simulink library "Susp_Components"  (R2026a)
settings: Solver=VariableStepAuto
undefined symbols (not defined in the file): clr_conn_links, clr_conn_rod, clr_link, clr_uaf, hp_in_f_ua, hp_out_f_ua, hp_shock_bot, hp_shock_botL, hp_shock_top, hp_shock_topL, hp_steerlink_out, hp_steerlink_outL, hp_upr_axle, hp_upr_axleL, hp_upr_drag, hp_upr_dragL, hp_wattsl_body, hp_wattsl_pivot, hp_wattsp_axle, hp_wattsu_body, hp_wattsu_pivot, hp_whl_ctr, hp_whl_ctrL, opc_conn_links, opc_conn_rod, opc_link, opc_uaf, radius_link, radius_uaf, size_conn_links, size_conn_rod, Susp, uaf_mass, upr_mass, Visual, wattsl_mass, wattsp_mass, wattsu_mass, X, Y, Z
libraries: sm_lib x32, Suspension_Utilities x10, Linkage_Shock x4, nesl_utility x3, $bdroot x2
(part 2 of 2)

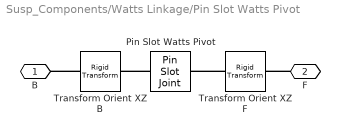
== system Susp_Components/Watts Linkage/Pin Slot Watts Pivot ==
  Pin Slot Watts Pivot : sm_lib/Joints/Pin Slot Joint  JointMode=Normal  CompositeWrenchDir=FollowerOnBase  CompositeWrenchFrame=BaseFrame  SenseConstraintForce=off  SenseConstraintTorque=off  SenseTotalForce=off  SenseTotalTorque=off  PxPositionTargetSpecify=off  PxPositionTargetPriority=High  PxPositionTargetValue=0  PxPositionTargetValueUnits=m  PxVelocityTargetSpecify=off  PxVelocityTargetPriority=High  PxVelocityTargetValue=0  PxVelocityTargetValueUnits=m/s  PxEquilibriumPosition=0  PxEquilibriumPositionUnits=m  PxSpringStiffness=0  PxSpringStiffnessUnits=N/m  PxDampingCoefficient=0  PxDampingCoefficientUnits=N/(m/s)  PxLowerLimitSpecify=off  PxLowerLimitBound=-1  PxLowerLimitBoundUnits=m  PxLowerLimitStiffness=1e6  PxLowerLimitStiffnessUnits=N/m  PxLowerLimitDamping=1e3  PxLowerLimitDampingUnits=N/(m/s)  PxLowerLimitTransitionRegionWidth=1e-4  PxLowerLimitTransitionRegionWidthUnits=m  PxUpperLimitSpecify=off  PxUpperLimitBound=1  PxUpperLimitBoundUnits=m  PxUpperLimitStiffness=1e6  PxUpperLimitStiffnessUnits=N/m  PxUpperLimitDamping=1e3  PxUpperLimitDampingUnits=N/(m/s)  PxUpperLimitTransitionRegionWidth=1e-4  PxUpperLimitTransitionRegionWidthUnits=m  PxTorqueActuationMode=NoTorque  PxMotionActuationMode=ComputedMotion  PxSensePosition=off  PxSenseVelocity=off  PxSenseAcceleration=off  PxSenseTorqueForce=off  PxSenseLowerLimitTorqueForce=off  PxSenseUpperLimitTorqueForce=off  RzPositionTargetSpecify=off  RzPositionTargetPriority=High  RzPositionTargetValue=0  RzPositionTargetValueUnits=deg  RzVelocityTargetSpecify=off  RzVelocityTargetPriority=High  RzVelocityTargetValue=0  RzVelocityTargetValueUnits=deg/s  RzEquilibriumPosition=0  RzEquilibriumPositionUnits=deg  RzSpringStiffness=0  RzSpringStiffnessUnits=N*m/deg  RzDampingCoefficient=0  RzDampingCoefficientUnits=N*m/(deg/s)  RzLowerLimitSpecify=off  RzLowerLimitBound=-90  RzLowerLimitBoundUnits=deg  RzLowerLimitStiffness=1e4  RzLowerLimitStiffnessUnits=N*m/deg  RzLowerLimitDamping=10  RzLowerLimitDampingUnits=N*m/(deg/s)  RzLowerLimitTransitionRegionWidth=0.1  RzLowerLimitTransitionRegionWidthUnits=deg  RzUpperLimitSpecify=off  RzUpperLimitBound=90  RzUpperLimitBoundUnits=deg  RzUpperLimitStiffness=1e4  RzUpperLimitStiffnessUnits=N*m/deg  RzUpperLimitDamping=10  RzUpperLimitDampingUnits=N*m/(deg/s)  RzUpperLimitTransitionRegionWidth=0.1  RzUpperLimitTransitionRegionWidthUnits=deg  RzTorqueActuationMode=NoTorque  RzMotionActuationMode=ComputedMotion  RzSensePosition=off  RzSenseVelocity=off  RzSenseAcceleration=off  RzSenseTorqueForce=off  RzSenseLowerLimitTorqueForce=off  RzSenseUpperLimitTorqueForce=off
  Transform Orient XZ B : sm_lib/Frames and Transforms/Rigid Transform  RotationMethod=AlignedAxes  FollAlignAxisA=+Z  BaseAlignAxisA=+X  FollAlignAxisB=+X  BaseAlignAxisB=+Y  RotationStandardAxis=+Z  RotationAngle=0.0  RotationAngleUnits=deg  RotationArbitraryAxis=[0 0 1]  RotationSequenceAxes=FollowerAxes  RotationSequence=XYX  RotationSequenceAngles=[0 0 0]  RotationSequenceAnglesUnits=deg  RotationMatrix=[1 0 0; 0 1 0; 0 0 1]  Quaternion=[1 0 0 0]  TranslationMethod=None  TranslationCartesianOffset=[0 0 0]  TranslationCartesianOffsetUnits=m  TranslationStandardAxis=+Z  TranslationStandardOffset=0  TranslationStandardOffsetUnits=m  TranslationROffset=0  TranslationROffsetUnits=m  TranslationThetaOffset=0  TranslationThetaOffsetUnits=deg  TranslationZOffset=0  TranslationZOffsetUnits=m
  Transform Orient XZ F : sm_lib/Frames and Transforms/Rigid Transform  RotationMethod=AlignedAxes  FollAlignAxisA=+Z  BaseAlignAxisA=+X  FollAlignAxisB=+X  BaseAlignAxisB=+Y  RotationStandardAxis=+Z  RotationAngle=0.0  RotationAngleUnits=deg  RotationArbitraryAxis=[0 0 1]  RotationSequenceAxes=FollowerAxes  RotationSequence=XYX  RotationSequenceAngles=[0 0 0]  RotationSequenceAnglesUnits=deg  RotationMatrix=[1 0 0; 0 1 0; 0 0 1]  Quaternion=[1 0 0 0]  TranslationMethod=None  TranslationCartesianOffset=[0 0 0]  TranslationCartesianOffsetUnits=m  TranslationStandardAxis=+Z  TranslationStandardOffset=0  TranslationStandardOffsetUnits=m  TranslationROffset=0  TranslationROffsetUnits=m  TranslationThetaOffset=0  TranslationThetaOffsetUnits=deg  TranslationZOffset=0  TranslationZOffsetUnits=m
  B : PMIOPort  Side=Left
  F : PMIOPort  Port=2  Side=Right
  connections:
  Transform Orient XZ F/RConn1 -- Pin Slot Watts Pivot/RConn1
  Pin Slot Watts Pivot/LConn1 -- Transform Orient XZ B/RConn1
  Transform Orient XZ B/LConn1 -- B/RConn1
  F/RConn1 -- Transform Orient XZ F/LConn1

== system Susp_Components/Watts Linkage/Universal Pivot Upper ==
  Transform Orient Z B : sm_lib/Frames and Transforms/Rigid Transform  RotationMethod=StandardAxis  FollAlignAxisA=+X  BaseAlignAxisA=+Y  FollAlignAxisB=+Y  BaseAlignAxisB=+Z  RotationStandardAxis=+X  RotationAngle=90  RotationAngleUnits=deg  RotationArbitraryAxis=[0 0 1]  RotationSequenceAxes=FollowerAxes  RotationSequence=XYX  RotationSequenceAngles=[0 0 0]  RotationSequenceAnglesUnits=deg  RotationMatrix=[1 0 0;0 1 0;0 0 1]  Quaternion=[1 0 0 0]  TranslationMethod=None  TranslationCartesianOffset=[0 0 0]  TranslationCartesianOffsetUnits=m  TranslationStandardAxis=+Z  TranslationStandardOffset=0  TranslationStandardOffsetUnits=m  TranslationROffset=0  TranslationROffsetUnits=m  TranslationThetaOffset=0  TranslationThetaOffsetUnits=deg  TranslationZOffset=0  TranslationZOffsetUnits=m
  Transform Orient Z F : sm_lib/Frames and Transforms/Rigid Transform  RotationMethod=StandardAxis  FollAlignAxisA=+X  BaseAlignAxisA=+Y  FollAlignAxisB=+Y  BaseAlignAxisB=+Z  RotationStandardAxis=+X  RotationAngle=90  RotationAngleUnits=deg  RotationArbitraryAxis=[0 0 1]  RotationSequenceAxes=FollowerAxes  RotationSequence=XYX  RotationSequenceAngles=[0 0 0]  RotationSequenceAnglesUnits=deg  RotationMatrix=[1 0 0;0 1 0;0 0 1]  Quaternion=[1 0 0 0]  TranslationMethod=None  TranslationCartesianOffset=[0 0 0]  TranslationCartesianOffsetUnits=m  TranslationStandardAxis=+Z  TranslationStandardOffset=0  TranslationStandardOffsetUnits=m  TranslationROffset=0  TranslationROffsetUnits=m  TranslationThetaOffset=0  TranslationThetaOffsetUnits=deg  TranslationZOffset=0  TranslationZOffsetUnits=m
  Universal Pivot Upper : sm_lib/Joints/Universal Joint  JointMode=Normal  CompositeWrenchDir=FollowerOnBase  CompositeWrenchFrame=BaseFrame  SenseConstraintForce=off  SenseConstraintTorque=off  SenseTotalForce=off  SenseTotalTorque=off  RxPositionTargetSpecify=off  RxPositionTargetPriority=High  RxPositionTargetValue=0  RxPositionTargetValueUnits=deg  RxVelocityTargetSpecify=off  RxVelocityTargetPriority=High  RxVelocityTargetValue=0  RxVelocityTargetValueUnits=deg/s  RxEquilibriumPosition=0  RxEquilibriumPositionUnits=deg  RxSpringStiffness=0  RxSpringStiffnessUnits=N*m/deg  RxDampingCoefficient=0  RxDampingCoefficientUnits=N*m/(deg/s)  RxLowerLimitSpecify=off  RxLowerLimitBound=-90  RxLowerLimitBoundUnits=deg  RxLowerLimitStiffness=1e4  RxLowerLimitStiffnessUnits=N*m/deg  RxLowerLimitDamping=10  RxLowerLimitDampingUnits=N*m/(deg/s)  RxLowerLimitTransitionRegionWidth=0.1  RxLowerLimitTransitionRegionWidthUnits=deg  RxUpperLimitSpecify=off  RxUpperLimitBound=90  RxUpperLimitBoundUnits=deg  RxUpperLimitStiffness=1e4  RxUpperLimitStiffnessUnits=N*m/deg  RxUpperLimitDamping=10  RxUpperLimitDampingUnits=N*m/(deg/s)  RxUpperLimitTransitionRegionWidth=0.1  RxUpperLimitTransitionRegionWidthUnits=deg  RxTorqueActuationMode=NoTorque  RxMotionActuationMode=ComputedMotion  RxSensePosition=off  RxSenseVelocity=off  RxSenseAcceleration=off  RxSenseTorqueForce=off  RxSenseLowerLimitTorqueForce=off  RxSenseUpperLimitTorqueForce=off  RyPositionTargetSpecify=off  RyPositionTargetPriority=High  RyPositionTargetValue=0  RyPositionTargetValueUnits=deg  RyVelocityTargetSpecify=off  RyVelocityTargetPriority=High  RyVelocityTargetValue=0  RyVelocityTargetValueUnits=deg/s  RyEquilibriumPosition=0  RyEquilibriumPositionUnits=deg  RySpringStiffness=0  RySpringStiffnessUnits=N*m/deg  RyDampingCoefficient=0  RyDampingCoefficientUnits=N*m/(deg/s)  RyLowerLimitSpecify=off  RyLowerLimitBound=-90  RyLowerLimitBoundUnits=deg  RyLowerLimitStiffness=1e4  RyLowerLimitStiffnessUnits=N*m/deg  RyLowerLimitDamping=10  RyLowerLimitDampingUnits=N*m/(deg/s)  RyLowerLimitTransitionRegionWidth=0.1  RyLowerLimitTransitionRegionWidthUnits=deg  RyUpperLimitSpecify=off  RyUpperLimitBound=90  RyUpperLimitBoundUnits=deg  RyUpperLimitStiffness=1e4  RyUpperLimitStiffnessUnits=N*m/deg  RyUpperLimitDamping=10  RyUpperLimitDampingUnits=N*m/(deg/s)  RyUpperLimitTransitionRegionWidth=0.1  RyUpperLimitTransitionRegionWidthUnits=deg  RyTorqueActuationMode=NoTorque  RyMotionActuationMode=ComputedMotion  RySensePosition=off  RySenseVelocity=off  RySenseAcceleration=off  RySenseTorqueForce=off  RySenseLowerLimitTorqueForce=off  RySenseUpperLimitTorqueForce=off
  B : PMIOPort  Side=Left
  F : PMIOPort  Port=2  Side=Right
  connections:
  Transform Orient Z B/RConn1 -- Universal Pivot Upper/LConn1
  Transform Orient Z B/LConn1 -- B/RConn1
  Transform Orient Z F/RConn1 -- Universal Pivot Upper/RConn1
  Transform Orient Z F/LConn1 -- F/RConn1

== system Susp_Components/Watts Linkage/Universal Watts Pivot Lower ==
  Transform Orient Z B : sm_lib/Frames and Transforms/Rigid Transform  RotationMethod=StandardAxis  FollAlignAxisA=+X  BaseAlignAxisA=+Y  FollAlignAxisB=+Y  BaseAlignAxisB=+Z  RotationStandardAxis=+X  RotationAngle=90  RotationAngleUnits=deg  RotationArbitraryAxis=[0 0 1]  RotationSequenceAxes=FollowerAxes  RotationSequence=XYX  RotationSequenceAngles=[0 0 0]  RotationSequenceAnglesUnits=deg  RotationMatrix=[1 0 0;0 1 0;0 0 1]  Quaternion=[1 0 0 0]  TranslationMethod=None  TranslationCartesianOffset=[0 0 0]  TranslationCartesianOffsetUnits=m  TranslationStandardAxis=+Z  TranslationStandardOffset=0  TranslationStandardOffsetUnits=m  TranslationROffset=0  TranslationROffsetUnits=m  TranslationThetaOffset=0  TranslationThetaOffsetUnits=deg  TranslationZOffset=0  TranslationZOffsetUnits=m
  Transform Orient Z F : sm_lib/Frames and Transforms/Rigid Transform  RotationMethod=StandardAxis  FollAlignAxisA=+X  BaseAlignAxisA=+Y  FollAlignAxisB=+Y  BaseAlignAxisB=+Z  RotationStandardAxis=+X  RotationAngle=90  RotationAngleUnits=deg  RotationArbitraryAxis=[0 0 1]  RotationSequenceAxes=FollowerAxes  RotationSequence=XYX  RotationSequenceAngles=[0 0 0]  RotationSequenceAnglesUnits=deg  RotationMatrix=[1 0 0;0 1 0;0 0 1]  Quaternion=[1 0 0 0]  TranslationMethod=None  TranslationCartesianOffset=[0 0 0]  TranslationCartesianOffsetUnits=m  TranslationStandardAxis=+Z  TranslationStandardOffset=0  TranslationStandardOffsetUnits=m  TranslationROffset=0  TranslationROffsetUnits=m  TranslationThetaOffset=0  TranslationThetaOffsetUnits=deg  TranslationZOffset=0  TranslationZOffsetUnits=m
  Universal Pivot Lower : sm_lib/Joints/Universal Joint  JointMode=Normal  CompositeWrenchDir=FollowerOnBase  CompositeWrenchFrame=BaseFrame  SenseConstraintForce=off  SenseConstraintTorque=off  SenseTotalForce=off  SenseTotalTorque=off  RxPositionTargetSpecify=off  RxPositionTargetPriority=High  RxPositionTargetValue=0  RxPositionTargetValueUnits=deg  RxVelocityTargetSpecify=off  RxVelocityTargetPriority=High  RxVelocityTargetValue=0  RxVelocityTargetValueUnits=deg/s  RxEquilibriumPosition=0  RxEquilibriumPositionUnits=deg  RxSpringStiffness=0  RxSpringStiffnessUnits=N*m/deg  RxDampingCoefficient=0  RxDampingCoefficientUnits=N*m/(deg/s)  RxLowerLimitSpecify=off  RxLowerLimitBound=-90  RxLowerLimitBoundUnits=deg  RxLowerLimitStiffness=1e4  RxLowerLimitStiffnessUnits=N*m/deg  RxLowerLimitDamping=10  RxLowerLimitDampingUnits=N*m/(deg/s)  RxLowerLimitTransitionRegionWidth=0.1  RxLowerLimitTransitionRegionWidthUnits=deg  RxUpperLimitSpecify=off  RxUpperLimitBound=90  RxUpperLimitBoundUnits=deg  RxUpperLimitStiffness=1e4  RxUpperLimitStiffnessUnits=N*m/deg  RxUpperLimitDamping=10  RxUpperLimitDampingUnits=N*m/(deg/s)  RxUpperLimitTransitionRegionWidth=0.1  RxUpperLimitTransitionRegionWidthUnits=deg  RxTorqueActuationMode=NoTorque  RxMotionActuationMode=ComputedMotion  RxSensePosition=off  RxSenseVelocity=off  RxSenseAcceleration=off  RxSenseTorqueForce=off  RxSenseLowerLimitTorqueForce=off  RxSenseUpperLimitTorqueForce=off  RyPositionTargetSpecify=off  RyPositionTargetPriority=High  RyPositionTargetValue=0  RyPositionTargetValueUnits=deg  RyVelocityTargetSpecify=off  RyVelocityTargetPriority=High  RyVelocityTargetValue=0  RyVelocityTargetValueUnits=deg/s  RyEquilibriumPosition=0  RyEquilibriumPositionUnits=deg  RySpringStiffness=0  RySpringStiffnessUnits=N*m/deg  RyDampingCoefficient=0  RyDampingCoefficientUnits=N*m/(deg/s)  RyLowerLimitSpecify=off  RyLowerLimitBound=-90  RyLowerLimitBoundUnits=deg  RyLowerLimitStiffness=1e4  RyLowerLimitStiffnessUnits=N*m/deg  RyLowerLimitDamping=10  RyLowerLimitDampingUnits=N*m/(deg/s)  RyLowerLimitTransitionRegionWidth=0.1  RyLowerLimitTransitionRegionWidthUnits=deg  RyUpperLimitSpecify=off  RyUpperLimitBound=90  RyUpperLimitBoundUnits=deg  RyUpperLimitStiffness=1e4  RyUpperLimitStiffnessUnits=N*m/deg  RyUpperLimitDamping=10  RyUpperLimitDampingUnits=N*m/(deg/s)  RyUpperLimitTransitionRegionWidth=0.1  RyUpperLimitTransitionRegionWidthUnits=deg  RyTorqueActuationMode=NoTorque  RyMotionActuationMode=ComputedMotion  RySensePosition=off  RySenseVelocity=off  RySenseAcceleration=off  RySenseTorqueForce=off  RySenseLowerLimitTorqueForce=off  RySenseUpperLimitTorqueForce=off
  B : PMIOPort  Side=Left
  F : PMIOPort  Port=2  Side=Right
  connections:
  Transform Orient Z F/LConn1 -- F/RConn1
  Transform Orient Z F/RConn1 -- Universal Pivot Lower/RConn1
  Transform Orient Z B/LConn1 -- B/RConn1
  Transform Orient Z B/RConn1 -- Universal Pivot Lower/LConn1

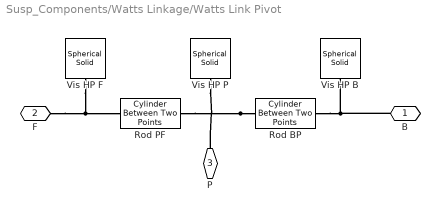
== system Susp_Components/Watts Linkage/Watts Link Pivot ==
  Rod BP : Suspension_Utilities/Cylinder Between Two Points  hp_b=hp_b.*[1 rhs_rod 1]  hp_f=hp_piv.*[1 rhs_rod 1]  Mass=rod_mass/2  clr_solid=clr_rod  opc_solid=opc_rod  rad_solid=radius_rod
  Rod PF : Suspension_Utilities/Cylinder Between Two Points  hp_b=hp_piv.*[1 rhs_rod 1]  hp_f=hp_f.*[1 rhs_rod 1]  Mass=rod_mass/2  clr_solid=clr_rod  opc_solid=opc_rod  rad_solid=radius_rod
  Vis HP B : sm_lib/Body Elements/Spherical Solid  SphereRadius=size_conn_rod  SphereRadiusUnits=m  ExportEntireGeometry=off  InertiaType=CalculateFromGeometry  BasedOnType=Density  Density=0  DensityUnits=kg/m^3  Mass=1  MassUnits=kg  CenterOfMass=[0 0 0]  CenterOfMassUnits=m  MomentsOfInertia=[1 1 1]  MomentsOfInertiaUnits=kg*m^2  ProductsOfInertia=[0 0 0]  ProductsOfInertiaUnits=kg*m^2  GraphicType=FromGeometry  MarkerShape=Sphere  MarkerSize=10  GraphicVisPropType=SimpleVisualProperties  GraphicDiffuseColor=clr_conn_rod  GraphicOpacity=opc_conn_rod  GraphicSpecularColor=[0.5 0.5 0.5 1.0]  GraphicAmbientColor=[0.15 0.15 0.15 1.0]  GraphicEmissiveColor=[0.0 0.0 0.0 1.0]  GraphicShininess=75  DoExposeReferenceFrame=on  SerializedFrames=<Frames/>
  Vis HP F : sm_lib/Body Elements/Spherical Solid  SphereRadius=size_conn_rod  SphereRadiusUnits=m  ExportEntireGeometry=off  InertiaType=CalculateFromGeometry  BasedOnType=Density  Density=0  DensityUnits=kg/m^3  Mass=1  MassUnits=kg  CenterOfMass=[0 0 0]  CenterOfMassUnits=m  MomentsOfInertia=[1 1 1]  MomentsOfInertiaUnits=kg*m^2  ProductsOfInertia=[0 0 0]  ProductsOfInertiaUnits=kg*m^2  GraphicType=FromGeometry  MarkerShape=Sphere  MarkerSize=10  GraphicVisPropType=SimpleVisualProperties  GraphicDiffuseColor=clr_conn_rod  GraphicOpacity=opc_conn_rod  GraphicSpecularColor=[0.5 0.5 0.5 1.0]  GraphicAmbientColor=[0.15 0.15 0.15 1.0]  GraphicEmissiveColor=[0.0 0.0 0.0 1.0]  GraphicShininess=75  DoExposeReferenceFrame=on  SerializedFrames=<Frames/>
  Vis HP P : sm_lib/Body Elements/Spherical Solid  SphereRadius=size_conn_rod  SphereRadiusUnits=m  ExportEntireGeometry=off  InertiaType=CalculateFromGeometry  BasedOnType=Density  Density=0  DensityUnits=kg/m^3  Mass=1  MassUnits=kg  CenterOfMass=[0 0 0]  CenterOfMassUnits=m  MomentsOfInertia=[1 1 1]  MomentsOfInertiaUnits=kg*m^2  ProductsOfInertia=[0 0 0]  ProductsOfInertiaUnits=kg*m^2  GraphicType=FromGeometry  MarkerShape=Sphere  MarkerSize=10  GraphicVisPropType=SimpleVisualProperties  GraphicDiffuseColor=clr_conn_rod  GraphicOpacity=opc_conn_rod  GraphicSpecularColor=[0.5 0.5 0.5 1.0]  GraphicAmbientColor=[0.15 0.15 0.15 1.0]  GraphicEmissiveColor=[0.0 0.0 0.0 1.0]  GraphicShininess=75  DoExposeReferenceFrame=on  SerializedFrames=<Frames/>
  B : PMIOPort  Side=Right
  F : PMIOPort  Port=2  Side=Left
  P : PMIOPort  Port=3  Side=Right
  connections:
  Rod BP/RConn1 -- Vis HP P/RConn1 -- P/RConn1 -- Rod PF/LConn1
  Vis HP F/RConn1 -- F/RConn1 -- Rod PF/RConn1
  B/RConn1 -- Rod BP/LConn1 -- Vis HP B/RConn1

== matlab function Susp_Components/Trailing Arm Bushing/MATLAB Function ==
  data: ang input; torque output; rate input
function torque = fcn(ang, rate)

    %t_damp   = damp_lookup(0.8*rate);
    %t_spring = spring_lookup(ang - 0.028769961);
    torque = -1*((880 + 97) + 2*(spring_lookup(ang - 0.028769961)) - (-0.3*rate^3 + 330*rate + 2*damp_lookup(0.8*rate)));
    
    
    function t_spring = spring_lookup(x)
    
        spring_x = [-0.1745329252
                    -0.1570796327
                    -0.1396263402
                    -0.1221730476
                    -0.1047197551
                    -8.72664626E-02
                    -6.981317008E-02
                    -5.235987756E-02
                    -3.490658504E-02
                    -1.745329252E-02
                    0.0
                    1.745329252E-02
                    3.490658504E-02
                    5.235987756E-02
                    6.981317008E-02
                    8.72664626E-02
                    0.1047197551
                    0.1221730476
                    0.1396263402
                    0.1570796327
                    0.1745329252];
        
        spring_t = [4807.6
                    3640.3569
                    2757.8432
                    2110.4923
                    1648.7376
                    1323.0125
                    1083.7504
                    881.3847
                    666.3488
                    389.0761
                    0.0
                    -389.0761
                    -666.3488
                    -881.3847
                    -1083.7504
                    -1323.0125
                    -1648.7376
                    -2110.4923
                    -2757.8432
                    -3640.3569
                    -4807.6];
    
        t_spring = interp1(spring_x, spring_t, x,'spline','extrap');
    
    end
    
    function t_damp = damp_lookup(v)
    
        damp_v = [-1.0
                  -0.9899497487
                  -0.9798994975
                  -0.9698492462
                  -0.959798995
                  -0.9497487437
                  -0.9396984925
                  -0.9296482412
                  -0.9195979899
                  -0.9095477387
                  -0.8994974874
                  -0.8894472362
                  -0.8793969849
                  -0.8693467337
                  -0.8592964824
                  -0.8492462312
                  -0.8391959799
                  -0.8291457286
                  -0.8190954774
                  -0.8090452261
                  -0.7989949749
                  -0.7889447236
                  -0.7788944724
                  -0.7688442211
                  -0.7587939698
                  -0.7487437186
                  -0.7386934673
                  -0.7286432161
                  -0.7185929648
                  -0.7085427136
                  -0.6984924623
                  -0.6884422111
                  -0.6783919598
                  -0.6683417085
                  -0.6582914573
                  -0.648241206
                  -0.6381909548
                  -0.6281407035
                  -0.6180904523
                  -0.608040201
                  -0.5979899497
                  -0.5879396985
                  -0.5778894472
                  -0.567839196
                  -0.5577889447
                  -0.5477386935
                  -0.5376884422
                  -0.527638191
                  -0.5175879397
                  -0.5075376884
                  -0.4974874372
                  -0.4874371859
                  -0.4773869347
                  -0.4673366834
                  -0.4572864322
                  -0.4472361809
                  -0.4371859296
                  -0.4271356784
                  -0.4170854271
                  -0.4070351759
                  -0.3969849246
                  -0.3869346734
                  -0.3768844221
                  -0.3668341709
                  -0.3567839196
                  -0.3467336683
                  -0.3366834171
                  -0.3266331658
                  -0.3165829146
                  -0.3065326633
                  -0.2964824121
                  -0.2864321608
                  -0.2763819095
                  -0.2663316583
                  -0.256281407
                  -0.2462311558
                  -0.2361809045
                  -0.2261306533
                  -0.216080402
                  -0.2060301508
                  -0.1959798995
                  -0.1859296482
                  -0.175879397
                  -0.1658291457
                  -0.1557788945
                  -0.1457286432
                  -0.135678392
                  -0.1256281407
                  -0.1155778894
                  -0.1055276382
                  -9.5477386935E-02
                  -8.5427135678E-02
                  -7.5376884422E-02
                  -6.5326633166E-02
                  -5.527638191E-02
                  -4.5226130653E-02
                  -3.5175879397E-02
                  -2.5125628141E-02
                  -1.5075376884E-02
                  -5.0251256281E-03
                  5.0251256281E-03
                  1.5075376884E-02
                  2.5125628141E-02
                  3.5175879397E-02
                  4.5226130653E-02
                  5.527638191E-02
                  6.5326633166E-02
                  7.5376884422E-02
                  8.5427135678E-02
                  9.5477386935E-02
                  0.1055276382
                  0.1155778894
                  0.1256281407
                  0.135678392
                  0.1457286432
                  0.1557788945
                  0.1658291457
                  0.175879397
                  0.1859296482
                  0.1959798995
                  0.2060301508
                  0.216080402
                  0.2261306533
                  0.2361809045
                  0.2462311558
                  0.256281407
                  0.2663316583
                  0.2763819095
                  0.2864321608
                  0.2964824121
                  0.3065326633
                  0.3165829146
                  0.3266331658
                  0.3366834171
                  0.3467336683
                  0.3567839196
                  0.3668341709
                  0.3768844221
                  0.3869346734
                  0.3969849246
                  0.4070351759
                  0.4170854271
                  0.4271356784
                  0.4371859296
                  0.4472361809
                  0.4572864322
                  0.4673366834
                  0.4773869347
                  0.4874371859
                  0.4974874372
                  0.5075376884
                  0.5175879397
                  0.527638191
                  0.5376884422
                  0.5477386935
                  0.5577889447
                  0.567839196
                  0.5778894472
                  0.5879396985
                  0.5979899497
                  0.608040201
                  0.6180904523
                  0.6281407035
                  0.6381909548
                  0.648241206
                  0.6582914573
                  0.6683417085
                  0.6783919598
                  0.6884422111
                  0.6984924623
                  0.7085427136
                  0.7185929648
                  0.7286432161
                  0.7386934673
                  0.7487437186
                  0.7587939698
                  0.7688442211
                  0.7788944724
                  0.7889447236
                  0.7989949749
                  0.8090452261
                  0.8190954774
                  0.8291457286
                  0.8391959799
                  0.8492462312
                  0.8592964824
                  0.8693467337
                  0.8793969849
                  0.8894472362
                  0.8994974874
                  0.9095477387
                  0.9195979899
                  0.9296482412
                  0.9396984925
                  0.9497487437
                  0.959798995
                  0.9698492462
                  0.9798994975
                  0.9899497487
                  1.0];
        
        
        damp_t = [51.2339934788
                  51.2492837167
                  51.2645802127
                  51.2798829681
                  51.2951919841
                  51.3105072622
                  51.3258288035
                  51.3411566093
                  51.3564906809
                  51.3718310196
                  51.3871776266
                  51.4025305033
                  51.4178896509
                  51.4332550707
                  51.448626764
                  51.4640047321
                  51.4793889762
                  51.4947794976
                  51.5101762977
                  51.5255793776
                  51.5409887387
                  51.5564043822
                  51.5718263095
                  51.5872545218
                  51.6026890204
                  51.6181298065
                  51.6335768815
                  51.6490302466
                  51.6644899031
                  51.6799558523
                  51.6954280955
                  51.710906634
                  51.7263914689
                  51.7418826017
                  51.7573800336
                  51.7728837658
                  51.7883937997
                  51.8039101366
                  51.8194327776
                  51.8349617242
                  51.8504969775
                  51.8660385389
                  51.8815864096
                  51.8971405909
                  51.9127010841
                  51.9282678905
                  51.9438410114
                  51.959420448
                  51.9750062016
                  51.9905982735
                  52.006196665
                  52.0218013773
                  52.0374124118
                  52.0530297697
                  52.0686534524
                  52.0842834609
                  52.0999197968
                  52.1155624612
                  52.1312114554
                  52.1468667807
                  52.1625284385
                  52.1781964298
                  52.1938707561
                  52.2095514187
                  52.2252384187
                  52.2409317576
                  52.2566314365
                  52.2723374567
                  52.2880498196
                  52.3037685264
                  52.3194935783
                  52.3352249768
                  52.3509627229
                  52.3667068182
                  52.3824572637
                  52.3982140608
                  52.4139772108
                  52.4297467149
                  52.4455225745
                  52.4613047907
                  52.477093365
                  52.4928882985
                  52.5086895926
                  52.5244972486
                  52.5403112676
                  52.556131651
                  52.5719584001
                  52.5877915162
                  52.6036310005
                  52.6194768543
                  52.6353290789
                  52.6511876756
                  52.6670526456
                  56.206528248
                  64.0018308282
                  71.4274786528
                  79.9533254136
                  91.6133237526
                  106.3720160593
                  136.9945941997
                  -136.9945941997
                  -106.3720160593
                  -91.6133237526
                  -79.9533254136
                  -71.4274786528
                  -64.0018308282
                  -56.206528248
                  -52.6670526456
                  -52.6511876756
                  -52.6353290789
                  -52.6194768543
                  -52.6036310005
                  -52.5877915162
                  -52.5719584001
                  -52.556131651
                  -52.5403112676
                  -52.5244972486
                  -52.5086895926
                  -52.4928882985
                  -52.477093365
                  -52.4613047907
                  -52.4455225745
                  -52.4297467149
                  -52.4139772108
                  -52.3982140608
                  -52.3824572637
                  -52.3667068182
                  -52.3509627229
                  -52.3352249768
                  -52.3194935783
                  -52.3037685264
                  -52.2880498196
                  -52.2723374567
                  -52.2566314365
                  -52.2409317576
                  -52.2252384187
                  -52.2095514187
                  -52.1938707561
                  -52.1781964298
                  -52.1625284385
                  -52.1468667807
                  -52.1312114554
                  -52.1155624612
                  -52.0999197968
                  -52.0842834609
                  -52.0686534524
                  -52.0530297697
                  -52.0374124118
                  -52.0218013773
                  -52.006196665
                  -51.9905982735
                  -51.9750062016
                  -51.959420448
                  -51.9438410114
                  -51.9282678905
                  -51.9127010841
                  -51.8971405909
                  -51.8815864096
                  -51.8660385389
                  -51.8504969775
                  -51.8349617242
                  -51.8194327776
                  -51.8039101366
                  -51.7883937997
                  -51.7728837658
                  -51.7573800336
                  -51.7418826017
                  -51.7263914689
                  -51.710906634
                  -51.6954280955
                  -51.6799558523
                  -51.6644899031
                  -51.6490302466
                  -51.6335768815
                  -51.6181298065
                  -51.6026890204
                  -51.5872545218
                  -51.5718263095
                  -51.5564043822
                  -51.5409887387
                  -51.5255793776
                  -51.5101762977
                  -51.4947794976
                  -51.4793889762
                  -51.4640047321
                  -51.448626764
                  -51.4332550707
                  -51.4178896509
                  -51.4025305033
                  -51.3871776266
                  -51.3718310196
                  -51.3564906809
                  -51.3411566093
                  -51.3258288035
                  -51.3105072622
                  -51.2951919841
                  -51.2798829681
                  -51.2645802127
                  -51.2492837167
                  -51.2339934788];
        
        t_damp = interp1(damp_v, damp_t, v,'spline','extrap');
    
    end

end
